simulink model "Evaporator_Simulink_MPC_expanded"  (R2025b)
settings: Solver=VariableStepAuto  StartTime=t0  StopTime=5000  RelTol=1e-3
values from neighbouring files (symbols this model uses):
  A_aug = [Ad,               zeros(n_states, n_outputs) ... (first row only)    [evaporator_MPC_expanded_0.m]
  Ad = sys_est_d.A    [evaporator_MPC_expanded_0.m]
  B_aug = [Bd ... (first row only)    [evaporator_MPC_expanded_0.m]
  Bd_est = sys_est_d.B    [evaporator_MPC_expanded_0.m]
  Cd = eye(3)    [evaporator_MPC_expanded_0.m]
  Dd_est = sys_est_d.D    [evaporator_MPC_expanded_0.m]
  L2_opt = xOpt(2)    [evaporator_MPC_expanded_0.m]
  P2_opt = xOpt(1)    [evaporator_MPC_expanded_0.m]
  Q_aug = diag([100, 1, 50, 10, 1, 10])    [evaporator_MPC_expanded_0.m]
  R_weight = eye(4) * 0.1    [evaporator_MPC_expanded_0.m]
  Ts = 0.5    [evaporator_MPC_expanded_0.m]
  u_lb = [0; 0; 1; 100] - u_mv_nom    [evaporator_MPC_expanded_0.m]
  u_mv_nom = [F2_opt; F3_opt; F200_opt; P100_opt]    [evaporator_MPC_expanded_0.m]
  u_ub = [20; 80; 380; 380] - u_mv_nom    [evaporator_MPC_expanded_0.m]
  X2_opt = xOpt(3)    [evaporator_MPC_expanded_0.m]
undefined symbols (not defined in the file or in its folder): DiscIntNeverNeededParam, Discrete, dist, Time
libraries: simulink x7, ctrlSharedLib x1
settings Model: Creator=maxen  LastModifiedBy=malcolmrenney

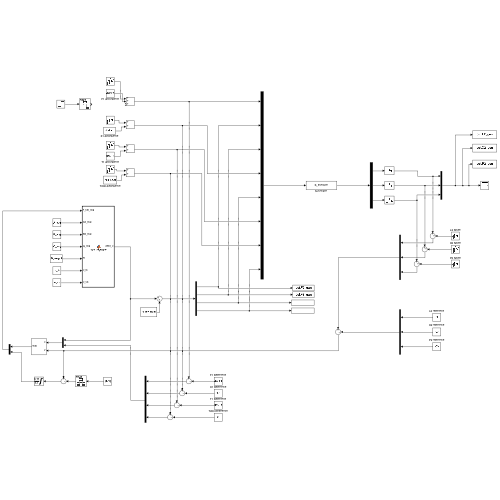
[thumbnail: Simulink's stored preview of the top-level diagram]
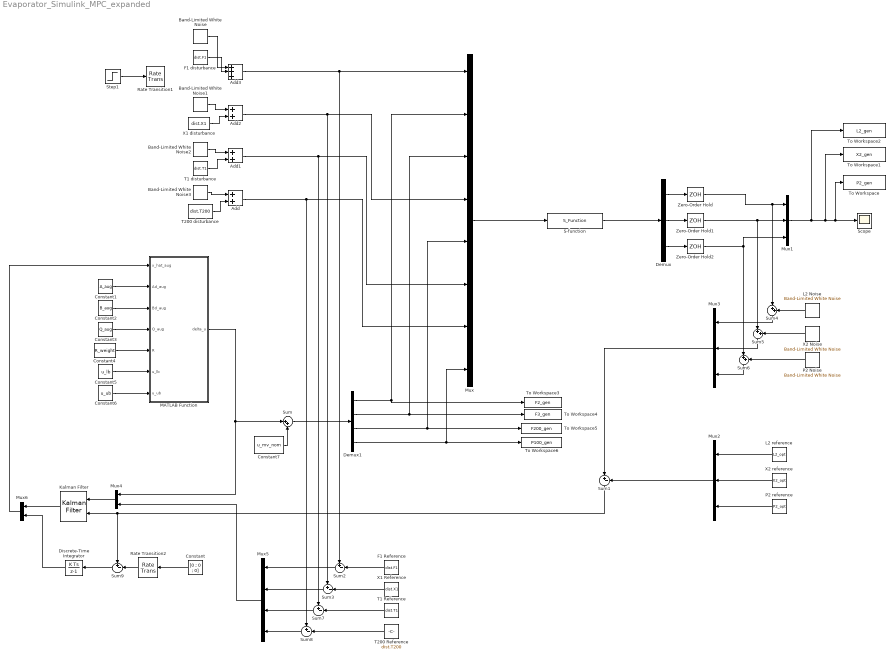
== system Evaporator_Simulink_MPC_expanded ==
  Add : Sum
  Add1 : Sum
  Add2 : Sum
  Add3 : Sum  Inputs=+++
  Band-Limited White Noise{,1..3} (4 alike) : simulink/Sources/Band-Limited White Noise  Cov=[0.1]  Ts=0.5  seed=[23341]
  Constant : Constant  Value=[0 ; 0 ; 0]
  Constant1 : Constant  Value=A_aug
  Constant2 : Constant  Value=B_aug
  Constant3 : Constant  Value=Q_aug
  Constant4 : Constant  Value=R_weight
  Constant5 : Constant  Value=u_lb
  Constant6 : Constant  Value=u_ub
  Constant7 : Constant  Value=u_mv_nom
  Demux : Demux  Outputs=3
  Demux1 : Demux
  Discrete-Time Integrator : DiscreteIntegrator  SampleTime=-1  LimitOutput=on  UpperSaturationLimit=0.5  LowerSaturationLimit=-0.5  ICPrevOutput=DiscIntNeverNeededParam  ICPrevScaledInput=DiscIntNeverNeededParam
  F1 Reference : Constant  Value=dist.F1
  F1 disturbance : Constant  Value=dist.F1
  Kalman Filter : ctrlSharedLib/Kalman Filter  TimeDomain=Discrete-Time  UseCurrentEstimator=on  ModelSource=LTI State-Space Variable  ModelSourceVariable=ss(Ad, Bd_est, Cd, Dd_est, Ts)  A=0.95  B=1  C=1  D=0  NumberOfStates=1  NumberOfInputs=1  NumberOfOutputs=1  InitialEstimateSource=Dialog  X0=0  P0=10  UseK=off  UseGH=off  NumberOfProcessNoiseInputs=1  G=1  TimeInvariantG=on  H=0  TimeInvariantH=on  Q=eye(3) * 0.01  TimeInvariantQ=on  R=eye(3) * 0.01  TimeInvariantR=on  N=0  TimeInvariantN=on  AddInputPort=on  AddEnablePort=off  OutputEstimatedY=off  OutputP=off  Ts=-1
  L2 Noise : simulink/Sources/Band-Limited White Noise  Cov=var_L  Ts=0.5  seed=[23341]
  L2 reference : Constant  Value=L2_opt
  MATLAB Function : MATLAB Function  TreatAsAtomicUnit=on
  Mux : Mux  Inputs=8
  Mux1 : Mux  Inputs=3
  Mux2 : Mux  Inputs=3
  Mux3 : Mux  Inputs=3
  Mux4 : Mux  Inputs=2
  Mux5 : Mux
  Mux6 : Mux  Inputs=2
  P2 Noise : simulink/Sources/Band-Limited White Noise  Cov=var_P  Ts=0.5  seed=[23341]
  P2 reference : Constant  Value=P2_opt
  Rate Transition1 : RateTransition
  Rate Transition2 : RateTransition
  "S-function " : S-Function  FunctionName=S_Function  Parameters=xinit, par  SFunctionDeploymentMode=off  EnableBusSupport=off
  Scope : Scope
      settings: ActiveDisplayYMinimum=-24.700190956168576  ActiveDisplayYMaximum=104.74258303555845
  Step1 : Step  Time=5000  After=0.5  SampleTime=0
  Sum{,4..6} (4 alike) : Sum  Inputs=|++
  Sum1 : Sum  Inputs=|+-
  Sum{2..3,7..9} (5 alike) : Sum  Inputs=+-|
  T1 Reference : Constant  Value=dist.T1
  T1 disturbance : Constant  Value=dist.T1
  T200 Reference : Constant  Value=dist.T200
  T200 disturbance : Constant  Value=dist.T200
  To Workspace : ToWorkspace  VariableName=P2_gen  SaveFormat=Timeseries  SampleTime=-1
  To Workspace1 : ToWorkspace  VariableName=X2_gen  SaveFormat=Timeseries  SampleTime=-1
  To Workspace2 : ToWorkspace  VariableName=L2_gen  SaveFormat=Timeseries  SampleTime=-1
  To Workspace3 : ToWorkspace  VariableName=F2_gen  SaveFormat=Timeseries  SampleTime=-1
  To Workspace4 : ToWorkspace  VariableName=F3_gen  SaveFormat=Timeseries  SampleTime=-1
  To Workspace5 : ToWorkspace  VariableName=F200_gen  SaveFormat=Timeseries  SampleTime=-1
  To Workspace6 : ToWorkspace  VariableName=P100_gen  SaveFormat=Timeseries  SampleTime=-1
  X1 Reference : Constant  Value=dist.X1
  X1 disturbance : Constant  Value=dist.X1
  X2 Noise : simulink/Sources/Band-Limited White Noise  Cov=var_X  Ts=0.5  seed=[23341]
  X2 reference : Constant  Value=X2_opt
  Zero-Order Hold : ZeroOrderHold  SampleTime=-1
  Zero-Order Hold1 : ZeroOrderHold  SampleTime=-1
  Zero-Order Hold2 : ZeroOrderHold  SampleTime=-1
  wires:
  Mux/1 -> "S-function "/1
  L2 reference/1 -> Mux2/1
  P2 reference/1 -> Mux2/3
  "S-function "/1 -> Demux/1
  Mux1/1 -> To Workspace2/1, To Workspace1/1, To Workspace/1, Scope/1
  Demux1/1 -> To Workspace3/1, Mux/2
  Demux1/2 -> To Workspace4/1, Mux/3
  Demux1/3 -> Mux/5, To Workspace5/1
  Demux1/4 -> To Workspace6/1, Mux/8
  L2 Noise/1 -> Sum4/2
  X2 Noise/1 -> Sum5/2
  P2 Noise/1 -> Sum6/2
  Sum4/1 -> Mux3/1
  Sum5/1 -> Mux3/2
  Sum6/1 -> Mux3/3
  MATLAB Function/1(delta_u) -> Mux4/1, Sum/1
  Sum/1 -> Demux1/1
  Constant7/1 -> Sum/2
  Constant2/1 -> MATLAB Function/3(Bd_aug)
  Constant1/1 -> MATLAB Function/2(Ad_aug)
  Constant6/1 -> MATLAB Function/7(u_ub)
  Constant5/1 -> MATLAB Function/6(u_lb)
  Constant4/1 -> MATLAB Function/5(R)
  Constant3/1 -> MATLAB Function/4(Q_aug)
  Sum1/1 -> Sum9/1, Kalman Filter/2
  Mux2/1 -> Sum1/2
  Mux3/1 -> Sum1/1
  F1 Reference/1 -> Sum2/2
  Sum2/1 -> Mux5/1
  X1 Reference/1 -> Sum3/2
  Sum3/1 -> Mux5/2
  T1 Reference/1 -> Sum7/2
  Sum7/1 -> Mux5/3
  T200 Reference/1 -> Sum8/2
  Sum8/1 -> Mux5/4
  Mux5/1 -> Mux4/2
  Band-Limited White Noise/1 -> Add3/1
  Band-Limited White Noise1/1 -> Add2/1
  X1 disturbance/1 -> Add2/2
  Band-Limited White Noise2/1 -> Add1/1
  T1 disturbance/1 -> Add1/2
  Band-Limited White Noise3/1 -> Add/1
  T200 disturbance/1 -> Add/2
  Add3/1 -> Mux/1, Sum2/1
  Add2/1 -> Mux/4, Sum3/1
  Add1/1 -> Sum7/1, Mux/6
  Add/1 -> Sum8/1, Mux/7
  Mux4/1 -> Kalman Filter/1
  Demux/1 -> Zero-Order Hold/1
  Zero-Order Hold/1 -> Sum4/1, Mux1/1
  Demux/3 -> Zero-Order Hold2/1
  Demux/2 -> Zero-Order Hold1/1
  Zero-Order Hold1/1 -> Sum5/1, Mux1/2
  Zero-Order Hold2/1 -> Sum6/1, Mux1/3
  Step1/1 -> Rate Transition1/1
  F1 disturbance/1 -> Add3/2
  Kalman Filter/1 -> Mux6/1
  Mux6/1 -> MATLAB Function/1(x_hat_aug)
  Discrete-Time Integrator/1 -> Mux6/2
  Sum9/1 -> Discrete-Time Integrator/1
  Rate Transition2/1 -> Sum9/2
  Constant/1 -> Rate Transition2/1
  X2 reference/1 -> Mux2/2

== matlab function Evaporator_Simulink_MPC_expanded/MATLAB Function ==
  data: x_hat_aug input; delta_u output; Ad_aug input; Bd_aug input; Q_aug input; R input; u_lb input; u_ub input
function delta_u = mpc_regulator(x_hat_aug, Ad_aug, Bd_aug, Q_aug, R, u_lb, u_ub)
    % 1. Pre-initialize variables
    delta_u = zeros(4, 1); 
    tmp = zeros(4, 1);     
    exitflag = 0;          
    x0 = zeros(4, 1); % Initial point for quadprog
    
    coder.extrinsic('quadprog', 'optimoptions');
    
    % --- QP Formulation ---
    H_raw = 2 * (Bd_aug' * Q_aug * Bd_aug + R);
    H = (H_raw + H_raw') / 2; % Force symmetry
    f = 2 * Bd_aug' * Q_aug * (Ad_aug * x_hat_aug);

    % --- Output Constraints (L2) ---
    B_L2 = Bd_aug(1, :); 
    L2_limit_min = -0.7; 
    L2_limit_max = 1.0;  

    A_ineq = [-B_L2; B_L2];
    b_ineq = [-(L2_limit_min - x_hat_aug(1)); (L2_limit_max - x_hat_aug(1))];

    % --- Solver Options ---
    % Switched to 'interior-point-convex' as it's often more robust in Simulink
    % and doesn't strictly require x0, but we provide it anyway.
    opts = optimoptions('quadprog', 'Algorithm', 'interior-point-convex', 'Display', 'off');

    % 2. Solve the optimization
    % Added x0 as the 9th argument
    [tmp, ~, exitflag] = quadprog(H, f, A_ineq, b_ineq, [], [], u_lb, u_ub, x0, opts);

    % 3. Assign result safely
    if exitflag > 0 
        delta_u = tmp;
    else
        % If infeasible, hold current valve positions (delta_u = 0)
        delta_u = zeros(4, 1); 
    end
end
